simulink model "ElevatorPlant_Storage_A"  (R2015b)
(part 8 of 8)

            state First_but_3
              en:
              BUT_1=BUT_TEMP;
              FIRST_BUT=false;
            (default) -> (junction 79574)
            (junction 79574) -> Emergency.Doors.Closing2.Button_detection.BUTTON_DOWN.Button_DOWN_1 [order 1] : [PD1]
            Emergency.Doors.Closing2.Button_detection.BUTTON_DOWN.Button_DOWN_1 -> (junction 79575)
            (junction 79575) -> Emergency.Doors.Closing2.Button_detection.BUTTON_DOWN.First_but_1 [order 1] : [FIRST_BUT && not(RPC1)]
            Emergency.Doors.Closing2.Button_detection.BUTTON_DOWN.First_but_1 -> (junction 79576)
            (junction 79574) -> (junction 79577) [order 2]
            (junction 79575) -> (junction 79578) [order 2]
            (junction 79576) -> (junction 79579)
            (junction 79578) -> (junction 79577)
            (junction 79579) -> (junction 79578)
            (junction 79577) -> (junction 79580)
            (junction 79580) -> Emergency.Doors.Closing2.Button_detection.BUTTON_DOWN.Button_DOWN_2 [order 1] : [PD2]
            Emergency.Doors.Closing2.Button_detection.BUTTON_DOWN.Button_DOWN_2 -> (junction 79581)
            (junction 79581) -> Emergency.Doors.Closing2.Button_detection.BUTTON_DOWN.First_but_2 [order 1] : [FIRST_BUT && not(RPC2)]
            Emergency.Doors.Closing2.Button_detection.BUTTON_DOWN.First_but_2 -> (junction 79582)
            (junction 79580) -> (junction 79583) [order 2]
            (junction 79581) -> (junction 79584) [order 2]
            (junction 79582) -> (junction 79585)
            (junction 79584) -> (junction 79583)
            (junction 79585) -> (junction 79584)
            (junction 79583) -> (junction 79586)
            (junction 79586) -> Emergency.Doors.Closing2.Button_detection.BUTTON_DOWN.Button_DOWN_3 [order 1] : [PD3]
            Emergency.Doors.Closing2.Button_detection.BUTTON_DOWN.Button_DOWN_3 -> (junction 79587)
            (junction 79587) -> Emergency.Doors.Closing2.Button_detection.BUTTON_DOWN.First_but_3 [order 1] : [FIRST_BUT && not(RPC3)]
            Emergency.Doors.Closing2.Button_detection.BUTTON_DOWN.First_but_3 -> (junction 79588)
            (junction 79586) -> (junction 79589) [order 2]
            (junction 79587) -> (junction 79590) [order 2]
            (junction 79588) -> (junction 79591)
            (junction 79590) -> (junction 79589)
            (junction 79591) -> (junction 79590)
          state BUTTON_CAR
            state Button_CAR_0
              en:
              BUTTON_CAR(1)=true;
              BUT_TEMP=0;
              LPC0=true;
              PUSHED=true;
              UPDATE=false;
              IN_LL=false; ET_LL=0;
            state First_but_0
              en:
              BUT_1=BUT_TEMP;
              FIRST_BUT=false;
            state Button_CAR_1
              en:
              BUTTON_CAR(2)=true;
              BUT_TEMP=1;
              LPC1=true;
              PUSHED=true;
              UPDATE=false;
              IN_LL=false; ET_LL=0;
            state First_but_1
              en:
              BUT_1=BUT_TEMP;
              FIRST_BUT=false;
            state Button_CAR_2
              en:
              BUTTON_CAR(3)=true;
              BUT_TEMP=2;
              LPC2=true;
              PUSHED=true;
              UPDATE=false;
              IN_LL=false; ET_LL=0;
            state First_but_2
              en:
              BUT_1=BUT_TEMP;
              FIRST_BUT=false;
            state Button_CAR_3
              en:
              BUTTON_CAR(4)=true;
              BUT_TEMP=3;
              LPC3=true;
              PUSHED=true;
              UPDATE=false;
              IN_LL=false; ET_LL=0;
            state First_but_3
              en:
              BUT_1=BUT_TEMP;
              FIRST_BUT=false;
            (default) -> (junction 79629)
            (junction 79629) -> Emergency.Doors.Closing2.Button_detection.BUTTON_CAR.Button_CAR_0 [order 1] : [P0]
            Emergency.Doors.Closing2.Button_detection.BUTTON_CAR.Button_CAR_0 -> (junction 79630)
            (junction 79630) -> Emergency.Doors.Closing2.Button_detection.BUTTON_CAR.First_but_0 [order 1] : [FIRST_BUT && not(RPC0)]
            Emergency.Doors.Closing2.Button_detection.BUTTON_CAR.First_but_0 -> (junction 79631)
            (junction 79629) -> (junction 79632) [order 2]
            (junction 79630) -> (junction 79633) [order 2]
            (junction 79631) -> (junction 79634)
            (junction 79633) -> (junction 79632)
            (junction 79634) -> (junction 79633)
            (junction 79632) -> (junction 79637)
            Emergency.Doors.Closing2.Button_detection.BUTTON_CAR.Button_CAR_1 -> (junction 79635)
            (junction 79635) -> Emergency.Doors.Closing2.Button_detection.BUTTON_CAR.First_but_1 [order 1] : [FIRST_BUT && not(RPC1)]
            Emergency.Doors.Closing2.Button_detection.BUTTON_CAR.First_but_1 -> (junction 79636)
            (junction 79635) -> (junction 79639) [order 2]
            (junction 79636) -> (junction 79640)
            (junction 79637) -> Emergency.Doors.Closing2.Button_detection.BUTTON_CAR.Button_CAR_1 [order 1] : [P1]
            (junction 79637) -> (junction 79638) [order 2]
            (junction 79639) -> (junction 79638)
            (junction 79640) -> (junction 79639)
            (junction 79638) -> (junction 79641)
            (junction 79641) -> Emergency.Doors.Closing2.Button_detection.BUTTON_CAR.Button_CAR_2 [order 1] : [P2]
            Emergency.Doors.Closing2.Button_detection.BUTTON_CAR.Button_CAR_2 -> (junction 79642)
            (junction 79642) -> Emergency.Doors.Closing2.Button_detection.BUTTON_CAR.First_but_2 [order 1] : [FIRST_BUT && not(RPC2)]
            Emergency.Doors.Closing2.Button_detection.BUTTON_CAR.First_but_2 -> (junction 79643)
            (junction 79641) -> (junction 79644) [order 2]
            (junction 79642) -> (junction 79645) [order 2]
            (junction 79643) -> (junction 79646)
            (junction 79645) -> (junction 79644)
            (junction 79646) -> (junction 79645)
            (junction 79644) -> (junction 79647)
            (junction 79647) -> Emergency.Doors.Closing2.Button_detection.BUTTON_CAR.Button_CAR_3 [order 1] : [P3]
            Emergency.Doors.Closing2.Button_detection.BUTTON_CAR.Button_CAR_3 -> (junction 79648)
            (junction 79648) -> Emergency.Doors.Closing2.Button_detection.BUTTON_CAR.First_but_3 [order 1] : [FIRST_BUT && not(RPC3)]
            Emergency.Doors.Closing2.Button_detection.BUTTON_CAR.First_but_3 -> (junction 79649)
            (junction 79647) -> (junction 79650) [order 2]
            (junction 79648) -> (junction 79651) [order 2]
            (junction 79649) -> (junction 79652)
            (junction 79651) -> (junction 79650)
            (junction 79652) -> (junction 79651)
          state BUTTON_UP
            state Button_UP_0
              en:
              BUTTON_UP(1)=true;
              BUT_TEMP=0;
              LPS0=true;
              PUSHED=true;
              UPDATE=false;
              IN_LL=false; ET_LL=0;
            state First_but_0
              en:
              BUT_1=BUT_TEMP;
              FIRST_BUT=false;
            state Button_UP_1
              en:
              BUTTON_UP(2)=true;
              BUT_TEMP=1;
              LPS1=true;
              PUSHED=true;
              UPDATE=false;
              IN_LL=false; ET_LL=0;
            state First_but_1
              en:
              BUT_1=BUT_TEMP;
              FIRST_BUT=false;
            state Button_UP_2
              en:
              BUTTON_UP(3)=true;
              BUT_TEMP=2;
              LPS2=true;
              PUSHED=true;
              UPDATE=false;
              IN_LL=false; ET_LL=0;
            state First_but_2
              en:
              BUT_1=BUT_TEMP;
              FIRST_BUT=false;
            (junction 79702) -> Emergency.Doors.Closing2.Button_detection.BUTTON_UP.Button_UP_0 [order 1] : [PS0]
            Emergency.Doors.Closing2.Button_detection.BUTTON_UP.Button_UP_0 -> (junction 79703)
            (junction 79703) -> Emergency.Doors.Closing2.Button_detection.BUTTON_UP.First_but_0 [order 1] : [FIRST_BUT && not(RPC0)]
            Emergency.Doors.Closing2.Button_detection.BUTTON_UP.First_but_0 -> (junction 79704)
            (default) -> (junction 79702)
            (junction 79702) -> (junction 79707) [order 2]
            (junction 79703) -> (junction 79705) [order 2]
            (junction 79704) -> (junction 79706)
            (junction 79706) -> (junction 79705)
            (junction 79705) -> (junction 79707)
            (junction 79707) -> (junction 79708)
            (junction 79708) -> Emergency.Doors.Closing2.Button_detection.BUTTON_UP.Button_UP_1 [order 1] : [PS1]
            Emergency.Doors.Closing2.Button_detection.BUTTON_UP.Button_UP_1 -> (junction 79709)
            (junction 79709) -> Emergency.Doors.Closing2.Button_detection.BUTTON_UP.First_but_1 [order 1] : [FIRST_BUT && not(RPC1)]
            Emergency.Doors.Closing2.Button_detection.BUTTON_UP.First_but_1 -> (junction 79710)
            (junction 79708) -> (junction 79711) [order 2]
            (junction 79709) -> (junction 79712) [order 2]
            (junction 79710) -> (junction 79713)
            (junction 79712) -> (junction 79711)
            (junction 79713) -> (junction 79712)
            (junction 79711) -> (junction 79715)
            Emergency.Doors.Closing2.Button_detection.BUTTON_UP.First_but_2 -> (junction 79714)
            (junction 79714) -> (junction 79719)
            (junction 79715) -> Emergency.Doors.Closing2.Button_detection.BUTTON_UP.Button_UP_2 [order 1] : [PS2]
            Emergency.Doors.Closing2.Button_detection.BUTTON_UP.Button_UP_2 -> (junction 79716)
            (junction 79716) -> Emergency.Doors.Closing2.Button_detection.BUTTON_UP.First_but_2 [order 1] : [FIRST_BUT && not(RPC2)]
            (junction 79715) -> (junction 79717) [order 2]
            (junction 79716) -> (junction 79718) [order 2]
            (junction 79718) -> (junction 79717)
            (junction 79719) -> (junction 79718)
          state Max_Min_assignment
            state Min_but
              en:
              BUTTON=MIN_BUT;
            state Max_but
              en:
              BUTTON=MAX_BUT;
            state First_but
              en:
              BUTTON=BUT_1;
            state Max_but1
              en:
              MAX_BUT=2;
            state Max_but2
              en:
              MAX_BUT=1;
            state Max_but3
              en:
              MAX_BUT=0;
            state Min_but1
              en:
              MIN_BUT=1;
            state Min_but2
              en:
              MIN_BUT=2;
            state Min_but3
              en:
              MIN_BUT=3;
            state MAX
              en:
              MAX_BUT=BUT_TEMP;
            state MIN
              en:
              MIN_BUT=BUT_TEMP;
            state Updating_button_0
              en:
              BUTTON=MAX_BUT;
            state Updating_button_1
              en:
              BUTTON=MIN_BUT;
            (junction 79757) -> Emergency.Doors.Closing2.Button_detection.Max_Min_assignment.Min_but [order 1] : [(MAX_BUT-FLOOR)>(FLOOR-MIN_BUT)]
            Emergency.Doors.Closing2.Button_detection.Max_Min_assignment.Min_but -> (junction 79758)
            (junction 79759) -> (junction 79757) [order 1] : [not(FLAG_STOP) && MOTION==2 && FLAG==3]
            (default) -> (junction 79759)
            (junction 79757) -> (junction 79760) [order 2]
            (junction 79758) -> (junction 79761)
            (junction 79759) -> (junction 79762) [order 2]
            (junction 79760) -> Emergency.Doors.Closing2.Button_detection.Max_Min_assignment.Max_but [order 1] : [(MAX_BUT-FLOOR)<(FLOOR-MIN_BUT)]
            Emergency.Doors.Closing2.Button_detection.Max_Min_assignment.Max_but -> (junction 79761)
            (junction 79760) -> Emergency.Doors.Closing2.Button_detection.Max_Min_assignment.First_but [order 2]
            (junction 79761) -> (junction 79764)
            Emergency.Doors.Closing2.Button_detection.Max_Min_assignment.First_but -> (junction 79763)
            (junction 79763) -> (junction 79762)
            (junction 79764) -> (junction 79763)
            (junction 79762) -> (junction 79765)
            (junction 79766) -> (junction 79767) [order 1] : [MOTION==0]
                | {MOTION=1;
                | UPDATE=true;}
            (junction 79767) -> Emergency.Doors.Closing2.Button_detection.Max_Min_assignment.Max_but1 [order 1] : [BUTTON_UP(2)]
            Emergency.Doors.Closing2.Button_detection.Max_Min_assignment.Max_but1 -> (junction 79768)
            (junction 79765) -> (junction 79766) [order 1] : [BUTTON==FLOOR && EXTEND]
                | {EXTEND=false;}
            (junction 79765) -> (junction 79779) [order 2]
            (junction 79766) -> (junction 79771) [order 2]
            (junction 79767) -> (junction 79769) [order 2]
            (junction 79768) -> (junction 79770)
            (junction 79769) -> Emergency.Doors.Closing2.Button_detection.Max_Min_assignment.Max_but2 [order 1] : [BUTTON_UP(1)]
            Emergency.Doors.Closing2.Button_detection.Max_Min_assignment.Max_but2 -> (junction 79770)
            (junction 79769) -> Emergency.Doors.Closing2.Button_detection.Max_Min_assignment.Max_but3 [order 2]
            (junction 79770) -> (junction 79773)
            Emergency.Doors.Closing2.Button_detection.Max_Min_assignment.Max_but3 -> (junction 79772)
            (junction 79772) -> (junction 79771)
            (junction 79773) -> (junction 79772)
            (junction 79771) -> (junction 79774)
            (junction 79774) -> (junction 79775) [order 1] : [MOTION==1]
                | {MOTION=0;
                | UPDATE=true;}
            (junction 79775) -> Emergency.Doors.Closing2.Button_detection.Max_Min_assignment.Min_but1 [order 1] : [BUTTON_DOWN(1)]
            Emergency.Doors.Closing2.Button_detection.Max_Min_assignment.Min_but1 -> (junction 79776)
            (junction 79774) -> (junction 79780) [order 2]
            (junction 79775) -> (junction 79777) [order 2]
            (junction 79776) -> (junction 79778)
            (junction 79777) -> Emergency.Doors.Closing2.Button_detection.Max_Min_assignment.Min_but2 [order 1] : [BUTTON_DOWN(2)]
            Emergency.Doors.Closing2.Button_detection.Max_Min_assignment.Min_but2 -> (junction 79778)
            (junction 79777) -> Emergency.Doors.Closing2.Button_detection.Max_Min_assignment.Min_but3 [order 2]
            (junction 79778) -> (junction 79782)
            Emergency.Doors.Closing2.Button_detection.Max_Min_assignment.Min_but3 -> (junction 79781)
            (junction 79780) -> (junction 79779)
            (junction 79781) -> (junction 79780)
            (junction 79782) -> (junction 79781)
            (junction 79779) -> (junction 79784)
            Emergency.Doors.Closing2.Button_detection.Max_Min_assignment.MAX -> (junction 79783)
            (junction 79784) -> (junction 79785) [order 1] : [PUSHED]
            (junction 79785) -> (junction 79786) [order 1] : [not(BUT_TEMP==FLOOR) || not(MOTION==2)]
            (junction 79786) -> Emergency.Doors.Closing2.Button_detection.Max_Min_assignment.MAX [order 1] : [MAX_BUT<BUT_TEMP && not(UPDATE)]
            (junction 79783) -> (junction 79788)
            (junction 79784) -> (junction 79798) [order 2]
            (junction 79785) -> (junction 79791) [order 2]
            (junction 79786) -> (junction 79787) [order 2]
            (junction 79788) -> (junction 79787)
            (junction 79787) -> (junction 79789)
            (junction 79789) -> Emergency.Doors.Closing2.Button_detection.Max_Min_assignment.MIN [order 1] : [MIN_BUT>BUT_TEMP && not(UPDATE)]
            Emergency.Doors.Closing2.Button_detection.Max_Min_assignment.MIN -> (junction 79790)
            (junction 79789) -> (junction 79792) [order 2]
            (junction 79790) -> (junction 79793)
            (junction 79792) -> (junction 79791)
            (junction 79793) -> (junction 79792)
            (junction 79791) -> (junction 79794)
            (junction 79794) -> Emergency.Doors.Closing2.Button_detection.Max_Min_assignment.Updating_button_0 [order 1] : [MOTION==0]
            Emergency.Doors.Closing2.Button_detection.Max_Min_assignment.Updating_button_0 -> (junction 79795)
            (junction 79794) -> (junction 79796) [order 2]
            (junction 79795) -> (junction 79797)
            (junction 79796) -> Emergency.Doors.Closing2.Button_detection.Max_Min_assignment.Updating_button_1 [order 1] : [MOTION==1]
            Emergency.Doors.Closing2.Button_detection.Max_Min_assignment.Updating_button_1 -> (junction 79797)
            (junction 79796) -> (junction 79799) [order 2]
            (junction 79797) -> (junction 79800)
            (junction 79799) -> (junction 79798)
            (junction 79800) -> (junction 79799)
          state GoTo_PositionControl
            en:
            BUTTON=BUT_TEMP;
            FLAG=2;
          state Emergency
            en:
            FLAG_EMG=true;
            FLAG=4;
          state Timer_EME
            state Set_tmr
              en:
              Q_EME=true;
            state Counting
              en:
              ET_EME= ET_EME + 1;
              Q_EME=false;
            state Set
              en:
              IN_EME=true;
              PT_EME=3;
            (junction 79890) -> Emergency.Doors.Closing2.Button_detection.Timer_EME.Set_tmr [order 1] : [ET_EME==PT_EME]
            Emergency.Doors.Closing2.Button_detection.Timer_EME.Set_tmr -> (junction 79891)
            Emergency.Doors.Closing2.Button_detection.Timer_EME.Counting -> (junction 79890)
            (junction 79890) -> (junction 79891) [order 2]
            (default) -> Emergency.Doors.Closing2.Button_detection.Timer_EME.Set
            Emergency.Doors.Closing2.Button_detection.Timer_EME.Set -> (junction 79892)
            (junction 79892) -> Emergency.Doors.Closing2.Button_detection.Timer_EME.Counting [order 1] : [ET_EME<PT_EME]
            (junction 79892) -> (junction 79891) [order 2]
          state Not_Emergency
            en:
            IN_EME=false;
            ET_EME=0;
          state SwitchingOFF_LEDs
            en:
            LPD3=false;
            LPD2=false;
            LPS2=false;
            LPD1=false;
            LPS1=false;
            LPS0=false;
          (default) -> (junction 79491)
          (junction 79491) -> (junction 79492) [order 1] : [FLAG==1 && not(PUSHED)]
              | {BUTTON=FLOOR;
              | BUT_TEMP=BUTTON;
              | BUT_1=FLOOR;}
          (junction 79492) -> Emergency.Doors.Closing2.Button_detection.Timer_LL [order 1] : [not(FLAG_STOP)]
          Emergency.Doors.Closing2.Button_detection.Save_energy -> (junction 79493)
          Emergency.Doors.Closing2.Button_detection.Timer_LL -> Emergency.Doors.Closing2.Button_detection.Save_energy
          (junction 79492) -> (junction 79495) [order 2]
          (junction 79491) -> (junction 79494) [order 2]
          (junction 79493) -> (junction 79496)
          (junction 79495) -> (junction 79494)
          (junction 79496) -> (junction 79495)
          (junction 79494) -> Emergency.Doors.Closing2.Button_detection.BUTTON_CAR
          Emergency.Doors.Closing2.Button_detection.BUTTON_UP -> Emergency.Doors.Closing2.Button_detection.BUTTON_DOWN
          Emergency.Doors.Closing2.Button_detection.BUTTON_DOWN -> Emergency.Doors.Closing2.Button_detection.Max_Min_assignment
          Emergency.Doors.Closing2.Button_detection.Max_Min_assignment -> (junction 79497)
          Emergency.Doors.Closing2.Button_detection.BUTTON_CAR -> Emergency.Doors.Closing2.Button_detection.BUTTON_UP
          (junction 79497) -> (junction 79499)
          (junction 79499) -> (junction 79498)
          (junction 79498) -> (junction 79501)
          Emergency.Doors.Closing2.Button_detection.GoTo_PositionControl -> (junction 79500)
          (junction 79501) -> (junction 79502) [order 1] : [FLAG==1]
          (junction 79502) -> Emergency.Doors.Closing2.Button_detection.GoTo_PositionControl [order 1] : [PUSHED]
          (junction 79500) -> (junction 79504)
          (junction 79501) -> (junction 79512) [order 2]
          (junction 79502) -> (junction 79503) [order 2]
          (junction 79504) -> (junction 79503)
          (junction 79503) -> (junction 79506)
          Emergency.Doors.Closing2.Button_detection.Emergency -> (junction 79505)
          (junction 79506) -> Emergency.Doors.Closing2.Button_detection.Timer_EME [order 1] : [STOP]
              | {IN_LL=false; ET_LL=0;FLAG=1;}
          Emergency.Doors.Closing2.Button_detection.Timer_EME -> (junction 79507)
          (junction 79507) -> Emergency.Doors.Closing2.Button_detection.Emergency [order 1] : [Q_EME]
          (junction 79505) -> (junction 79509)
          (junction 79506) -> Emergency.Doors.Closing2.Button_detection.Not_Emergency [order 2]
          (junction 79507) -> (junction 79508) [order 2]
          (junction 79509) -> (junction 79508)
          (junction 79508) -> (junction 79511)
          Emergency.Doors.Closing2.Button_detection.Not_Emergency -> (junction 79511)
          Emergency.Doors.Closing2.Button_detection.SwitchingOFF_LEDs -> (junction 79510)
          (junction 79511) -> Emergency.Doors.Closing2.Button_detection.SwitchingOFF_LEDs [order 1] : [FLAG_STOP && FLAG==2]
          (junction 79510) -> (junction 79514)
          (junction 79511) -> (junction 79513) [order 2]
          (junction 79513) -> (junction 79512)
          (junction 79514) -> (junction 79513)
        state Extending
          en:
          EXTEND=true;
        state Stop_Closing
          en:
          CP2=false;
          FLAG_OD=false;
          OBS=false;
          ET_cl=0;
          IN_cl=false;
        state GoTo_PositionControl
          en: FLAG=2;
        state GoTo_BUttonDetection
          en:
          MOTION=2;
          MAX_BUT=0;
          MIN_BUT=3;
          PUSHED=false;
          FIRST_BUT=true;
          FLAG=1;
          UPDATE=false;
        state Closing1
          en:CP2=true;
        state Stop_Closing1
          en:CP2=false;
        Emergency.Doors.Closing2.Reset -> Emergency.Doors.Closing2.Timer_close
        (default) -> (junction 79402)
        (junction 79402) -> Emergency.Doors.Closing2.Reset [order 1] : [not(FLAG==0) && not(FLAG==4)]
        Emergency.Doors.Closing2.Timer_close -> (junction 79403)
        (junction 79403) -> Emergency.Doors.Closing2.Closing [order 1] : [not(PC2)]
        Emergency.Doors.Closing2.Button_detection -> (junction 79404)
        Emergency.Doors.Closing2.Closing -> Emergency.Doors.Closing2.Button_detection
        (junction 79402) -> (junction 79412) [order 2]
        (junction 79403) -> (junction 79405) [order 2]
        (junction 79404) -> (junction 79410)
        (junction 79405) -> Emergency.Doors.Closing2.Extending [order 1] : [BUTTON==FLOOR]
        (junction 79405) -> (junction 79407) [order 2]
        Emergency.Doors.Closing2.Extending -> (junction 79406)
        (junction 79406) -> (junction 79407)
        (junction 79407) -> Emergency.Doors.Closing2.Stop_Closing
        Emergency.Doors.Closing2.Stop_Closing -> (junction 79408)
        (junction 79408) -> Emergency.Doors.Closing2.GoTo_PositionControl [order 2]
        (junction 79408) -> Emergency.Doors.Closing2.GoTo_BUttonDetection [order 1] : [not(BUTTON_CAR(1) || BUTTON_CAR(2) || BUTTON_CAR(3) || BUTTON_CAR(4) || BUTTON_UP(1) || BUTTON_UP(2) || BUTTON_UP(3) || BUTTON_DOWN(2) || BUTTON_DOWN(3) || BUTTON_DOWN(4))]
        Emergency.Doors.Closing2.GoTo_PositionControl -> (junction 79409)
        Emergency.Doors.Closing2.GoTo_BUttonDetection -> (junction 79409)
        (junction 79409) -> (junction 79410)
        (junction 79410) -> (junction 79411)
        (junction 79411) -> (junction 79413)
        (junction 79412) -> Emergency.Doors.Closing2.Closing1 [order 1] : [not(PC2)]
        Emergency.Doors.Closing2.Closing1 -> (junction 79413)
        (junction 79412) -> Emergency.Doors.Closing2.Stop_Closing1 [order 2]
        Emergency.Doors.Closing2.Stop_Closing1 -> (junction 79413)
      state Closing3
        state Reset
          state Reset_0
            en:
            LPS0=false;
            BUTTON_CAR(1)=false;
            BUTTON_UP(1)=false;
          state Reset_1
            en:
            LPS1=false;
            LPD1=false;
            BUTTON_CAR(2)=false;
            BUTTON_UP(2)=false;
            BUTTON_DOWN(2)=false;
          state Reset_2
            en:
            LPS2=false;
            LPD2=false;
            BUTTON_CAR(3)=false;
            BUTTON_UP(3)=false;
            BUTTON_DOWN(3)=false;
          state Reset_3
            en:
            LPD3=false;
            BUTTON_CAR(4)=false;
            BUTTON_DOWN(4)=false;
          (default) -> (junction 79953)
          (junction 79953) -> Emergency.Doors.Closing3.Reset.Reset_0 [order 1] : [FLOOR==0]
          Emergency.Doors.Closing3.Reset.Reset_0 -> (junction 79954)
          (junction 79953) -> (junction 79955) [order 2]
          (junction 79954) -> (junction 79956)
          (junction 79955) -> Emergency.Doors.Closing3.Reset.Reset_1 [order 1] : [FLOOR==1]
          Emergency.Doors.Closing3.Reset.Reset_1 -> (junction 79956)
          (junction 79955) -> (junction 79957) [order 2]
          (junction 79956) -> (junction 79958)
          (junction 79957) -> Emergency.Doors.Closing3.Reset.Reset_2 [order 1] : [FLOOR==2]
          Emergency.Doors.Closing3.Reset.Reset_2 -> (junction 79958)
          (junction 79957) -> (junction 79959) [order 2]
          (junction 79958) -> (junction 79960)
          (junction 79959) -> Emergency.Doors.Closing3.Reset.Reset_3 [order 1] : [FLOOR==3]
          Emergency.Doors.Closing3.Reset.Reset_3 -> (junction 79960)
          (junction 79959) -> (junction 79961) [order 2]
          (junction 79960) -> (junction 79962)
          (junction 79962) -> (junction 79961)
        state Timer_close
          state Set_tmr
            en: Q_cl=true;
          state Set
            en:PT_cl=5;
            IN_cl=true;
          state Counting
            en:ET_cl = ET_cl + 1;
            Q_cl=false;
          (junction 79986) -> Emergency.Doors.Closing3.Timer_close.Set_tmr [order 1] : [ET_cl==PT_cl]
          Emergency.Doors.Closing3.Timer_close.Set_tmr -> (junction 79987)
          (default) -> Emergency.Doors.Closing3.Timer_close.Set
          Emergency.Doors.Closing3.Timer_close.Counting -> (junction 79986)
          (junction 79986) -> (junction 79987) [order 2]
          Emergency.Doors.Closing3.Timer_close.Set -> (junction 79988)
          (junction 79988) -> Emergency.Doors.Closing3.Timer_close.Counting [order 1] : [ET_cl<PT_cl]
          (junction 79988) -> (junction 79987) [order 2]
        state Closing
          en: CP2=Q_cl;
        state Button_detection
          state Save_energy
            en:
            LL=not(Q_LL);
          state Timer_LL
            state Set_tmr
              en:
              Q_LL=true;
            state Counting
              en:
              ET_LL= ET_LL + 1;
              Q_LL=false;
            state Set
              en:
              IN_LL=true;
              PT_LL=10;
            (junction 80070) -> Emergency.Doors.Closing3.Button_detection.Timer_LL.Set_tmr [order 1] : [ET_LL==PT_LL]
            Emergency.Doors.Closing3.Button_detection.Timer_LL.Set_tmr -> (junction 80071)
            Emergency.Doors.Closing3.Button_detection.Timer_LL.Counting -> (junction 80070)
            (junction 80070) -> (junction 80071) [order 2]
            (default) -> Emergency.Doors.Closing3.Button_detection.Timer_LL.Set
            Emergency.Doors.Closing3.Button_detection.Timer_LL.Set -> (junction 80072)
            (junction 80072) -> Emergency.Doors.Closing3.Button_detection.Timer_LL.Counting [order 1] : [ET_LL<PT_LL]
            (junction 80072) -> (junction 80071) [order 2]
          state BUTTON_DOWN
            state Button_DOWN_1
              en:
              BUTTON_DOWN(2)=true;
              BUT_TEMP=1;
              LPD1=true;
              PUSHED=true;
              UPDATE=false;
              IN_LL=false; ET_LL=0;
            state First_but_1
              en:
              BUT_1=BUT_TEMP;
              FIRST_BUT=false;
            state Button_DOWN_2
              en:
              BUTTON_DOWN(3)=true;
              BUT_TEMP=2;
              LPD2=true;
              PUSHED=true;
              UPDATE=false;
              IN_LL=false; ET_LL=0;
            state First_but_2
              en:
              BUT_1=BUT_TEMP;
              FIRST_BUT=false;
            state Button_DOWN_3
              en:
              BUTTON_DOWN(4)=true;
              BUT_TEMP=3;
              LPD3=true;
              PUSHED=true;
              UPDATE=false;
              IN_LL=false; ET_LL=0;
            state First_but_3
              en:
              BUT_1=BUT_TEMP;
              FIRST_BUT=false;
            (default) -> (junction 80085)
            (junction 80085) -> Emergency.Doors.Closing3.Button_detection.BUTTON_DOWN.Button_DOWN_1 [order 1] : [PD1]
            Emergency.Doors.Closing3.Button_detection.BUTTON_DOWN.Button_DOWN_1 -> (junction 80086)
            (junction 80086) -> Emergency.Doors.Closing3.Button_detection.BUTTON_DOWN.First_but_1 [order 1] : [FIRST_BUT && not(RPC1)]
            Emergency.Doors.Closing3.Button_detection.BUTTON_DOWN.First_but_1 -> (junction 80087)
            (junction 80085) -> (junction 80088) [order 2]
            (junction 80086) -> (junction 80089) [order 2]
            (junction 80087) -> (junction 80090)
            (junction 80089) -> (junction 80088)
            (junction 80090) -> (junction 80089)
            (junction 80088) -> (junction 80091)
            (junction 80091) -> Emergency.Doors.Closing3.Button_detection.BUTTON_DOWN.Button_DOWN_2 [order 1] : [PD2]
            Emergency.Doors.Closing3.Button_detection.BUTTON_DOWN.Button_DOWN_2 -> (junction 80092)
            (junction 80092) -> Emergency.Doors.Closing3.Button_detection.BUTTON_DOWN.First_but_2 [order 1] : [FIRST_BUT && not(RPC2)]
            Emergency.Doors.Closing3.Button_detection.BUTTON_DOWN.First_but_2 -> (junction 80093)
            (junction 80091) -> (junction 80094) [order 2]
            (junction 80092) -> (junction 80095) [order 2]
            (junction 80093) -> (junction 80096)
            (junction 80095) -> (junction 80094)
            (junction 80096) -> (junction 80095)
            (junction 80094) -> (junction 80097)
            (junction 80097) -> Emergency.Doors.Closing3.Button_detection.BUTTON_DOWN.Button_DOWN_3 [order 1] : [PD3]
            Emergency.Doors.Closing3.Button_detection.BUTTON_DOWN.Button_DOWN_3 -> (junction 80098)
            (junction 80098) -> Emergency.Doors.Closing3.Button_detection.BUTTON_DOWN.First_but_3 [order 1] : [FIRST_BUT && not(RPC3)]
            Emergency.Doors.Closing3.Button_detection.BUTTON_DOWN.First_but_3 -> (junction 80099)
            (junction 80097) -> (junction 80100) [order 2]
            (junction 80098) -> (junction 80101) [order 2]
            (junction 80099) -> (junction 80102)
            (junction 80101) -> (junction 80100)
            (junction 80102) -> (junction 80101)
          state BUTTON_CAR
            state Button_CAR_0
              en:
              BUTTON_CAR(1)=true;
              BUT_TEMP=0;
              LPC0=true;
              PUSHED=true;
              UPDATE=false;
              IN_LL=false; ET_LL=0;
            state First_but_0
              en:
              BUT_1=BUT_TEMP;
              FIRST_BUT=false;
            state Button_CAR_1
              en:
              BUTTON_CAR(2)=true;
              BUT_TEMP=1;
              LPC1=true;
              PUSHED=true;
              UPDATE=false;
              IN_LL=false; ET_LL=0;
            state First_but_1
              en:
              BUT_1=BUT_TEMP;
              FIRST_BUT=false;
            state Button_CAR_2
              en:
              BUTTON_CAR(3)=true;
              BUT_TEMP=2;
              LPC2=true;
              PUSHED=true;
              UPDATE=false;
              IN_LL=false; ET_LL=0;
            state First_but_2
              en:
              BUT_1=BUT_TEMP;
              FIRST_BUT=false;
            state Button_CAR_3
              en:
              BUTTON_CAR(4)=true;
              BUT_TEMP=3;
              LPC3=true;
              PUSHED=true;
              UPDATE=false;
              IN_LL=false; ET_LL=0;
            state First_but_3
              en:
              BUT_1=BUT_TEMP;
              FIRST_BUT=false;
            (default) -> (junction 80140)
            (junction 80140) -> Emergency.Doors.Closing3.Button_detection.BUTTON_CAR.Button_CAR_0 [order 1] : [P0]
            Emergency.Doors.Closing3.Button_detection.BUTTON_CAR.Button_CAR_0 -> (junction 80141)
            (junction 80141) -> Emergency.Doors.Closing3.Button_detection.BUTTON_CAR.First_but_0 [order 1] : [FIRST_BUT && not(RPC0)]
            Emergency.Doors.Closing3.Button_detection.BUTTON_CAR.First_but_0 -> (junction 80142)
            (junction 80140) -> (junction 80143) [order 2]
            (junction 80141) -> (junction 80144) [order 2]
            (junction 80142) -> (junction 80145)
            (junction 80144) -> (junction 80143)
            (junction 80145) -> (junction 80144)
            (junction 80143) -> (junction 80148)
            Emergency.Doors.Closing3.Button_detection.BUTTON_CAR.Button_CAR_1 -> (junction 80146)
            (junction 80146) -> Emergency.Doors.Closing3.Button_detection.BUTTON_CAR.First_but_1 [order 1] : [FIRST_BUT && not(RPC1)]
            Emergency.Doors.Closing3.Button_detection.BUTTON_CAR.First_but_1 -> (junction 80147)
            (junction 80146) -> (junction 80150) [order 2]
            (junction 80147) -> (junction 80151)
            (junction 80148) -> Emergency.Doors.Closing3.Button_detection.BUTTON_CAR.Button_CAR_1 [order 1] : [P1]
            (junction 80148) -> (junction 80149) [order 2]
            (junction 80150) -> (junction 80149)
            (junction 80151) -> (junction 80150)
            (junction 80149) -> (junction 80152)
            (junction 80152) -> Emergency.Doors.Closing3.Button_detection.BUTTON_CAR.Button_CAR_2 [order 1] : [P2]
            Emergency.Doors.Closing3.Button_detection.BUTTON_CAR.Button_CAR_2 -> (junction 80153)
            (junction 80153) -> Emergency.Doors.Closing3.Button_detection.BUTTON_CAR.First_but_2 [order 1] : [FIRST_BUT && not(RPC2)]
            Emergency.Doors.Closing3.Button_detection.BUTTON_CAR.First_but_2 -> (junction 80154)
            (junction 80152) -> (junction 80155) [order 2]
            (junction 80153) -> (junction 80156) [order 2]
            (junction 80154) -> (junction 80157)
            (junction 80156) -> (junction 80155)
            (junction 80157) -> (junction 80156)
            (junction 80155) -> (junction 80158)
            (junction 80158) -> Emergency.Doors.Closing3.Button_detection.BUTTON_CAR.Button_CAR_3 [order 1] : [P3]
            Emergency.Doors.Closing3.Button_detection.BUTTON_CAR.Button_CAR_3 -> (junction 80159)
            (junction 80159) -> Emergency.Doors.Closing3.Button_detection.BUTTON_CAR.First_but_3 [order 1] : [FIRST_BUT && not(RPC3)]
            Emergency.Doors.Closing3.Button_detection.BUTTON_CAR.First_but_3 -> (junction 80160)
            (junction 80158) -> (junction 80161) [order 2]
            (junction 80159) -> (junction 80162) [order 2]
            (junction 80160) -> (junction 80163)
            (junction 80162) -> (junction 80161)
            (junction 80163) -> (junction 80162)
          state BUTTON_UP
            state Button_UP_0
              en:
              BUTTON_UP(1)=true;
              BUT_TEMP=0;
              LPS0=true;
              PUSHED=true;
              UPDATE=false;
              IN_LL=false; ET_LL=0;
            state First_but_0
              en:
              BUT_1=BUT_TEMP;
              FIRST_BUT=false;
            state Button_UP_1
              en:
              BUTTON_UP(2)=true;
              BUT_TEMP=1;
              LPS1=true;
              PUSHED=true;
              UPDATE=false;
              IN_LL=false; ET_LL=0;
            state First_but_1
              en:
              BUT_1=BUT_TEMP;
              FIRST_BUT=false;
            state Button_UP_2
              en:
              BUTTON_UP(3)=true;
              BUT_TEMP=2;
              LPS2=true;
              PUSHED=true;
              UPDATE=false;
              IN_LL=false; ET_LL=0;
            state First_but_2
              en:
              BUT_1=BUT_TEMP;
              FIRST_BUT=false;
            (junction 80213) -> Emergency.Doors.Closing3.Button_detection.BUTTON_UP.Button_UP_0 [order 1] : [PS0]
            Emergency.Doors.Closing3.Button_detection.BUTTON_UP.Button_UP_0 -> (junction 80214)
            (junction 80214) -> Emergency.Doors.Closing3.Button_detection.BUTTON_UP.First_but_0 [order 1] : [FIRST_BUT && not(RPC0)]
            Emergency.Doors.Closing3.Button_detection.BUTTON_UP.First_but_0 -> (junction 80215)
            (default) -> (junction 80213)
            (junction 80213) -> (junction 80218) [order 2]
            (junction 80214) -> (junction 80216) [order 2]
            (junction 80215) -> (junction 80217)
            (junction 80217) -> (junction 80216)
            (junction 80216) -> (junction 80218)
            (junction 80218) -> (junction 80219)
            (junction 80219) -> Emergency.Doors.Closing3.Button_detection.BUTTON_UP.Button_UP_1 [order 1] : [PS1]
            Emergency.Doors.Closing3.Button_detection.BUTTON_UP.Button_UP_1 -> (junction 80220)
            (junction 80220) -> Emergency.Doors.Closing3.Button_detection.BUTTON_UP.First_but_1 [order 1] : [FIRST_BUT && not(RPC1)]
            Emergency.Doors.Closing3.Button_detection.BUTTON_UP.First_but_1 -> (junction 80221)
            (junction 80219) -> (junction 80222) [order 2]
            (junction 80220) -> (junction 80223) [order 2]
            (junction 80221) -> (junction 80224)
            (junction 80223) -> (junction 80222)
            (junction 80224) -> (junction 80223)
            (junction 80222) -> (junction 80226)
            Emergency.Doors.Closing3.Button_detection.BUTTON_UP.First_but_2 -> (junction 80225)
            (junction 80225) -> (junction 80230)
            (junction 80226) -> Emergency.Doors.Closing3.Button_detection.BUTTON_UP.Button_UP_2 [order 1] : [PS2]
            Emergency.Doors.Closing3.Button_detection.BUTTON_UP.Button_UP_2 -> (junction 80227)
            (junction 80227) -> Emergency.Doors.Closing3.Button_detection.BUTTON_UP.First_but_2 [order 1] : [FIRST_BUT && not(RPC2)]
            (junction 80226) -> (junction 80228) [order 2]
            (junction 80227) -> (junction 80229) [order 2]
            (junction 80229) -> (junction 80228)
            (junction 80230) -> (junction 80229)
          state Max_Min_assignment
            state Min_but
              en:
              BUTTON=MIN_BUT;
            state Max_but
              en:
              BUTTON=MAX_BUT;
            state First_but
              en:
              BUTTON=BUT_1;
            state Max_but1
              en:
              MAX_BUT=2;
            state Max_but2
              en:
              MAX_BUT=1;
            state Max_but3
              en:
              MAX_BUT=0;
            state Min_but1
              en:
              MIN_BUT=1;
            state Min_but2
              en:
              MIN_BUT=2;
            state Min_but3
              en:
              MIN_BUT=3;
            state MAX
              en:
              MAX_BUT=BUT_TEMP;
            state MIN
              en:
              MIN_BUT=BUT_TEMP;
            state Updating_button_0
              en:
              BUTTON=MAX_BUT;
            state Updating_button_1
              en:
              BUTTON=MIN_BUT;
            (junction 80268) -> Emergency.Doors.Closing3.Button_detection.Max_Min_assignment.Min_but [order 1] : [(MAX_BUT-FLOOR)>(FLOOR-MIN_BUT)]
            Emergency.Doors.Closing3.Button_detection.Max_Min_assignment.Min_but -> (junction 80269)
            (junction 80270) -> (junction 80268) [order 1] : [not(FLAG_STOP) && MOTION==2 && FLAG==3]
            (default) -> (junction 80270)
            (junction 80268) -> (junction 80271) [order 2]
            (junction 80269) -> (junction 80272)
            (junction 80270) -> (junction 80273) [order 2]
            (junction 80271) -> Emergency.Doors.Closing3.Button_detection.Max_Min_assignment.Max_but [order 1] : [(MAX_BUT-FLOOR)<(FLOOR-MIN_BUT)]
            Emergency.Doors.Closing3.Button_detection.Max_Min_assignment.Max_but -> (junction 80272)
            (junction 80271) -> Emergency.Doors.Closing3.Button_detection.Max_Min_assignment.First_but [order 2]
            (junction 80272) -> (junction 80275)
            Emergency.Doors.Closing3.Button_detection.Max_Min_assignment.First_but -> (junction 80274)
            (junction 80274) -> (junction 80273)
            (junction 80275) -> (junction 80274)
            (junction 80273) -> (junction 80276)
            (junction 80277) -> (junction 80278) [order 1] : [MOTION==0]
                | {MOTION=1;
                | UPDATE=true;}
            (junction 80278) -> Emergency.Doors.Closing3.Button_detection.Max_Min_assignment.Max_but1 [order 1] : [BUTTON_UP(2)]
            Emergency.Doors.Closing3.Button_detection.Max_Min_assignment.Max_but1 -> (junction 80279)
            (junction 80276) -> (junction 80277) [order 1] : [BUTTON==FLOOR && EXTEND]
                | {EXTEND=false;}
            (junction 80276) -> (junction 80290) [order 2]
            (junction 80277) -> (junction 80282) [order 2]
            (junction 80278) -> (junction 80280) [order 2]
            (junction 80279) -> (junction 80281)
            (junction 80280) -> Emergency.Doors.Closing3.Button_detection.Max_Min_assignment.Max_but2 [order 1] : [BUTTON_UP(1)]
            Emergency.Doors.Closing3.Button_detection.Max_Min_assignment.Max_but2 -> (junction 80281)
            (junction 80280) -> Emergency.Doors.Closing3.Button_detection.Max_Min_assignment.Max_but3 [order 2]
            (junction 80281) -> (junction 80284)
            Emergency.Doors.Closing3.Button_detection.Max_Min_assignment.Max_but3 -> (junction 80283)
            (junction 80283) -> (junction 80282)
            (junction 80284) -> (junction 80283)
            (junction 80282) -> (junction 80285)
            (junction 80285) -> (junction 80286) [order 1] : [MOTION==1]
                | {MOTION=0;
                | UPDATE=true;}
            (junction 80286) -> Emergency.Doors.Closing3.Button_detection.Max_Min_assignment.Min_but1 [order 1] : [BUTTON_DOWN(1)]
            Emergency.Doors.Closing3.Button_detection.Max_Min_assignment.Min_but1 -> (junction 80287)
            (junction 80285) -> (junction 80291) [order 2]
            (junction 80286) -> (junction 80288) [order 2]
            (junction 80287) -> (junction 80289)
            (junction 80288) -> Emergency.Doors.Closing3.Button_detection.Max_Min_assignment.Min_but2 [order 1] : [BUTTON_DOWN(2)]
            Emergency.Doors.Closing3.Button_detection.Max_Min_assignment.Min_but2 -> (junction 80289)
            (junction 80288) -> Emergency.Doors.Closing3.Button_detection.Max_Min_assignment.Min_but3 [order 2]
            (junction 80289) -> (junction 80293)
            Emergency.Doors.Closing3.Button_detection.Max_Min_assignment.Min_but3 -> (junction 80292)
            (junction 80291) -> (junction 80290)
            (junction 80292) -> (junction 80291)
            (junction 80293) -> (junction 80292)
            (junction 80290) -> (junction 80295)
            Emergency.Doors.Closing3.Button_detection.Max_Min_assignment.MAX -> (junction 80294)
            (junction 80295) -> (junction 80296) [order 1] : [PUSHED]
            (junction 80296) -> (junction 80297) [order 1] : [not(BUT_TEMP==FLOOR) || not(MOTION==2)]
            (junction 80297) -> Emergency.Doors.Closing3.Button_detection.Max_Min_assignment.MAX [order 1] : [MAX_BUT<BUT_TEMP && not(UPDATE)]
            (junction 80294) -> (junction 80299)
            (junction 80295) -> (junction 80309) [order 2]
            (junction 80296) -> (junction 80302) [order 2]
            (junction 80297) -> (junction 80298) [order 2]
            (junction 80299) -> (junction 80298)
            (junction 80298) -> (junction 80300)
            (junction 80300) -> Emergency.Doors.Closing3.Button_detection.Max_Min_assignment.MIN [order 1] : [MIN_BUT>BUT_TEMP && not(UPDATE)]
            Emergency.Doors.Closing3.Button_detection.Max_Min_assignment.MIN -> (junction 80301)
            (junction 80300) -> (junction 80303) [order 2]
            (junction 80301) -> (junction 80304)
            (junction 80303) -> (junction 80302)
            (junction 80304) -> (junction 80303)
            (junction 80302) -> (junction 80305)
            (junction 80305) -> Emergency.Doors.Closing3.Button_detection.Max_Min_assignment.Updating_button_0 [order 1] : [MOTION==0]
            Emergency.Doors.Closing3.Button_detection.Max_Min_assignment.Updating_button_0 -> (junction 80306)
            (junction 80305) -> (junction 80307) [order 2]
            (junction 80306) -> (junction 80308)
            (junction 80307) -> Emergency.Doors.Closing3.Button_detection.Max_Min_assignment.Updating_button_1 [order 1] : [MOTION==1]
            Emergency.Doors.Closing3.Button_detection.Max_Min_assignment.Updating_button_1 -> (junction 80308)
            (junction 80307) -> (junction 80310) [order 2]
            (junction 80308) -> (junction 80311)
            (junction 80310) -> (junction 80309)
            (junction 80311) -> (junction 80310)
          state GoTo_PositionControl
            en:
            BUTTON=BUT_TEMP;
            FLAG=2;
          state Emergency
            en:
            FLAG_EMG=true;
            FLAG=4;
          state Timer_EME
            state Set_tmr
              en:
              Q_EME=true;
            state Counting
              en:
              ET_EME= ET_EME + 1;
              Q_EME=false;
            state Set
              en:
              IN_EME=true;
              PT_EME=3;
            (junction 80401) -> Emergency.Doors.Closing3.Button_detection.Timer_EME.Set_tmr [order 1] : [ET_EME==PT_EME]
            Emergency.Doors.Closing3.Button_detection.Timer_EME.Set_tmr -> (junction 80402)
            Emergency.Doors.Closing3.Button_detection.Timer_EME.Counting -> (junction 80401)
            (junction 80401) -> (junction 80402) [order 2]
            (default) -> Emergency.Doors.Closing3.Button_detection.Timer_EME.Set
            Emergency.Doors.Closing3.Button_detection.Timer_EME.Set -> (junction 80403)
            (junction 80403) -> Emergency.Doors.Closing3.Button_detection.Timer_EME.Counting [order 1] : [ET_EME<PT_EME]
            (junction 80403) -> (junction 80402) [order 2]
          state Not_Emergency
            en:
            IN_EME=false;
            ET_EME=0;
          state SwitchingOFF_LEDs
            en:
            LPD3=false;
            LPD2=false;
            LPS2=false;
            LPD1=false;
            LPS1=false;
            LPS0=false;
          (default) -> (junction 80002)
          (junction 80002) -> (junction 80003) [order 1] : [FLAG==1 && not(PUSHED)]
              | {BUTTON=FLOOR;
              | BUT_TEMP=BUTTON;
              | BUT_1=FLOOR;}
          (junction 80003) -> Emergency.Doors.Closing3.Button_detection.Timer_LL [order 1] : [not(FLAG_STOP)]
          Emergency.Doors.Closing3.Button_detection.Save_energy -> (junction 80004)
          Emergency.Doors.Closing3.Button_detection.Timer_LL -> Emergency.Doors.Closing3.Button_detection.Save_energy
          (junction 80003) -> (junction 80006) [order 2]
          (junction 80002) -> (junction 80005) [order 2]
          (junction 80004) -> (junction 80007)
          (junction 80006) -> (junction 80005)
          (junction 80007) -> (junction 80006)
          (junction 80005) -> Emergency.Doors.Closing3.Button_detection.BUTTON_CAR
          Emergency.Doors.Closing3.Button_detection.BUTTON_UP -> Emergency.Doors.Closing3.Button_detection.BUTTON_DOWN
          Emergency.Doors.Closing3.Button_detection.BUTTON_DOWN -> Emergency.Doors.Closing3.Button_detection.Max_Min_assignment
          Emergency.Doors.Closing3.Button_detection.Max_Min_assignment -> (junction 80008)
          Emergency.Doors.Closing3.Button_detection.BUTTON_CAR -> Emergency.Doors.Closing3.Button_detection.BUTTON_UP
          (junction 80008) -> (junction 80010)
          (junction 80010) -> (junction 80009)
          (junction 80009) -> (junction 80012)
          Emergency.Doors.Closing3.Button_detection.GoTo_PositionControl -> (junction 80011)
          (junction 80012) -> (junction 80013) [order 1] : [FLAG==1]
          (junction 80013) -> Emergency.Doors.Closing3.Button_detection.GoTo_PositionControl [order 1] : [PUSHED]
          (junction 80011) -> (junction 80015)
          (junction 80012) -> (junction 80023) [order 2]
          (junction 80013) -> (junction 80014) [order 2]
          (junction 80015) -> (junction 80014)
          (junction 80014) -> (junction 80017)
          Emergency.Doors.Closing3.Button_detection.Emergency -> (junction 80016)
          (junction 80017) -> Emergency.Doors.Closing3.Button_detection.Timer_EME [order 1] : [STOP]
              | {IN_LL=false; ET_LL=0;FLAG=1;}
          Emergency.Doors.Closing3.Button_detection.Timer_EME -> (junction 80018)
          (junction 80018) -> Emergency.Doors.Closing3.Button_detection.Emergency [order 1] : [Q_EME]
          (junction 80016) -> (junction 80020)
          (junction 80017) -> Emergency.Doors.Closing3.Button_detection.Not_Emergency [order 2]
          (junction 80018) -> (junction 80019) [order 2]
          (junction 80020) -> (junction 80019)
          (junction 80019) -> (junction 80022)
          Emergency.Doors.Closing3.Button_detection.Not_Emergency -> (junction 80022)
          Emergency.Doors.Closing3.Button_detection.SwitchingOFF_LEDs -> (junction 80021)
          (junction 80022) -> Emergency.Doors.Closing3.Button_detection.SwitchingOFF_LEDs [order 1] : [FLAG_STOP && FLAG==2]
          (junction 80021) -> (junction 80025)
          (junction 80022) -> (junction 80024) [order 2]
          (junction 80024) -> (junction 80023)
          (junction 80025) -> (junction 80024)
        state Extending
          en:
          EXTEND=true;
        state Stop_Closing
          en:
          CP2=false;
          FLAG_OD=false;
          OBS=false;
          ET_cl=0;
          IN_cl=false;
        state GoTo_PositionControl
          en: FLAG=2;
        state GoTo_BUttonDetection
          en:
          MOTION=2;
          MAX_BUT=0;
          MIN_BUT=3;
          PUSHED=false;
          FIRST_BUT=true;
          FLAG=1;
          UPDATE=false;
        state Closing1
          en:CP2=true;
        state Stop_Closing1
          en:CP2=false;
        Emergency.Doors.Closing3.Reset -> Emergency.Doors.Closing3.Timer_close
        (default) -> (junction 79913)
        (junction 79913) -> Emergency.Doors.Closing3.Reset [order 1] : [not(FLAG==0) && not(FLAG==4)]
        Emergency.Doors.Closing3.Timer_close -> (junction 79914)
        (junction 79914) -> Emergency.Doors.Closing3.Closing [order 1] : [not(PC2)]
        Emergency.Doors.Closing3.Button_detection -> (junction 79915)
        Emergency.Doors.Closing3.Closing -> Emergency.Doors.Closing3.Button_detection
        (junction 79913) -> (junction 79923) [order 2]
        (junction 79914) -> (junction 79916) [order 2]
        (junction 79915) -> (junction 79921)
        (junction 79916) -> Emergency.Doors.Closing3.Extending [order 1] : [BUTTON==FLOOR]
        (junction 79916) -> (junction 79918) [order 2]
        Emergency.Doors.Closing3.Extending -> (junction 79917)
        (junction 79917) -> (junction 79918)
        (junction 79918) -> Emergency.Doors.Closing3.Stop_Closing
        Emergency.Doors.Closing3.Stop_Closing -> (junction 79919)
        (junction 79919) -> Emergency.Doors.Closing3.GoTo_PositionControl [order 2]
        (junction 79919) -> Emergency.Doors.Closing3.GoTo_BUttonDetection [order 1] : [not(BUTTON_CAR(1) || BUTTON_CAR(2) || BUTTON_CAR(3) || BUTTON_CAR(4) || BUTTON_UP(1) || BUTTON_UP(2) || BUTTON_UP(3) || BUTTON_DOWN(2) || BUTTON_DOWN(3) || BUTTON_DOWN(4))]
        Emergency.Doors.Closing3.GoTo_PositionControl -> (junction 79920)
        Emergency.Doors.Closing3.GoTo_BUttonDetection -> (junction 79920)
        (junction 79920) -> (junction 79921)
        (junction 79921) -> (junction 79922)
        (junction 79922) -> (junction 79924)
        (junction 79923) -> Emergency.Doors.Closing3.Closing1 [order 1] : [not(PC2)]
        Emergency.Doors.Closing3.Closing1 -> (junction 79924)
        (junction 79923) -> Emergency.Doors.Closing3.Stop_Closing1 [order 2]
        Emergency.Doors.Closing3.Stop_Closing1 -> (junction 79924)
      FLOOR_0 -> Emergency.Doors.Opening0
      (junction 15604) -> (junction 15603) [order 1] : [(SWITCH || FLAG_EMG || FLAG_BO) && (RPC0 || RPC1 || RPC2 || RPC3)]
      (junction 15603) -> FLOOR_0 [order 1] : [FLOOR==0]
      Emergency.Doors.Opening0 -> (junction 36735)
      (default) -> (junction 15604)
      (junction 15604) -> (junction 36752) [order 2]
      (junction 15603) -> (junction 36727) [order 2]
      (junction 36735) -> (junction 36737)
      FLOOR_1 -> Emergency.Doors.Opening1
      (junction 36727) -> FLOOR_1 [order 1] : [FLOOR==1]
      Emergency.Doors.Opening1 -> (junction 36737)
      (junction 36727) -> (junction 36730) [order 2]
      (junction 36737) -> (junction 36741)
      FLOOR_2 -> Emergency.Doors.Opening2
      (junction 36730) -> FLOOR_2 [order 1] : [FLOOR==2]
      Emergency.Doors.Opening2 -> (junction 36741)
      (junction 36730) -> (junction 36732) [order 2]
      (junction 36741) -> (junction 36744)
      FLOOR_3 -> Emergency.Doors.Opening3
      Emergency.Doors.Opening3 -> (junction 36744)
      (junction 36732) -> FLOOR_3 [order 1] : [FLOOR==3]
      (junction 36744) -> (junction 36749)
      (junction 36732) -> (junction 36747) [order 2]
      (junction 36747) -> (junction 36752)
      (junction 36749) -> (junction 36747)
      (junction 36752) -> (junction 36755)
      (junction 36755) -> (junction 15605) [order 1] : [not(BO) && FLAG_OD && not(FLAG_EMG)]
      (junction 15605) -> Emergency.Doors.Closing0 [order 1] : [FLOOR==0]
      Emergency.Doors.Closing0 -> (junction 36764)
      (junction 36755) -> (junction 36780) [order 2]
      (junction 15605) -> (junction 36757) [order 2]
      (junction 36764) -> (junction 36766)
      (junction 36757) -> Emergency.Doors.Closing1 [order 1] : [FLOOR==1]
      Emergency.Doors.Closing1 -> (junction 36766)
      (junction 36757) -> (junction 36759) [order 2]
      (junction 36766) -> (junction 36767)
      Emergency.Doors.Closing2 -> (junction 36767)
      (junction 36759) -> Emergency.Doors.Closing2 [order 1] : [FLOOR==2]
      (junction 36767) -> (junction 36768)
      (junction 36759) -> (junction 36761) [order 2]
      (junction 36761) -> Emergency.Doors.Closing3 [order 1] : [FLOOR==3]
      Emergency.Doors.Closing3 -> (junction 36768)
      (junction 36761) -> (junction 36763) [order 2]
      (junction 36768) -> (junction 36769)
      (junction 36763) -> (junction 36780)
      (junction 36769) -> (junction 36763)
    state Timer_EME_OFF
      state Set_tmr
        en: Q_EME_OFF=true;
      state Counting
        en:ET_EME_OFF = ET_EME_OFF + 1;
        Q_EME_OFF=false;
      state Set
        en:PT_EME_OFF=3;
        IN_EME_OFF=true;
      (junction 16326) -> Emergency.Timer_EME_OFF.Set_tmr [order 1] : [ET_EME_OFF==PT_EME_OFF]
      Emergency.Timer_EME_OFF.Set_tmr -> (junction 16327)
      Emergency.Timer_EME_OFF.Counting -> (junction 16326)
      (junction 16326) -> (junction 16327) [order 2]
      (default) -> Emergency.Timer_EME_OFF.Set
      Emergency.Timer_EME_OFF.Set -> (junction 16328)
      (junction 16328) -> Emergency.Timer_EME_OFF.Counting [order 1] : [ET_EME_OFF<PT_EME_OFF]
      (junction 16328) -> (junction 16327) [order 2]
    state NOT_EME
      en:
      FLAG_EMG=false;
    state KEEP_EME
      en:
      IN_EME_OFF=false;
      ET_EME_OFF=0;
    state NOT_BO
      en:
      FLAG_BO=false;
    state EME_FINISH
      en:
      FLAG=1;
      LPS0=false; LPS1=false;
      LPD1=false; LPS2=false;
      LPD2=false; LPD3=false;
      OBS=false; FLAG_OD=false;
      IN_cl=false; ET_cl=0;
      IN_EME=false; ET_EME=0;
      IN_EME_OFF=false; ET_EME_OFF=0;
      FIRST=true; FLAG_REC=false;
      PUSHED=false;
      MAX_BUT=0; MIN_BUT=3;
    (junction 36672) -> BLK_Eme [order 1] : [FLAG_EMG]
    (default) -> (junction 36672)
    (junction 36672) -> (junction 36674) [order 2]
    BLK_Eme -> (junction 36675)
    (junction 36674) -> (junction 36675)
    (junction 36675) -> REC [order 1] : [FLAG_REC && BO]
    (junction 36675) -> (junction 36682) [order 2]
    REC -> (junction 36681)
    (junction 36682) -> (junction 36681)
    (junction 36681) -> FIRST [order 1] : [FIRST]
    (junction 36681) -> (junction 36687) [order 2]
    FIRST -> (junction 36686)
    (junction 36687) -> (junction 36686)
    (junction 36686) -> Emergency.Replacing [order 1] : [not(RPC0) && not(RPC1) && not(RPC2) && not(RPC3)]
    (junction 36686) -> Emergency.Replaced [order 2]
    Emergency.Replacing -> (junction 36692)
    Emergency.Replaced -> (junction 36691)
    Doors -> (junction 36697)
    (junction 36691) -> Doors
    (junction 36692) -> (junction 36691)
    (junction 36697) -> (junction 36699)
    (junction 36699) -> (junction 15583) [order 1] : [((not(BO) && not(FLAG_REC)) || FLAG_EMG) && not(FIRE)]
    (junction 15583) -> Timer_EME_OFF [order 1] : [STOP && (PA0 || PA1|| PA2 || PA3)]
    Timer_EME_OFF -> (junction 36701)
    (junction 36701) -> NOT_EME [order 1] : [Q_EME_OFF]
    (junction 36699) -> (junction 36711) [order 2]
    (junction 15583) -> KEEP_EME [order 2]
    (junction 36701) -> (junction 36703) [order 2]
    NOT_EME -> (junction 36705)
    KEEP_EME -> (junction 36708)
    (junction 36708) -> (junction 36711)
    (junction 36703) -> (junction 36708)
    (junction 36705) -> (junction 36703)
    (junction 36711) -> (junction 36714)
    (junction 36714) -> NOT_BO [order 1] : [(PA0 || PA1 || PA2 || PA3) && not(BO)]
    (junction 36714) -> (junction 36719) [order 2]
    NOT_BO -> (junction 36716)
    (junction 36719) -> (junction 36716)
    (junction 36716) -> EME_FINISH [order 1] : [(RPC0 || RPC1 || RPC2 || RPC3) && (PC0 && PC1 && PC2 && PC3) && not(FLAG_EMG) && not (BO)]
    (junction 36716) -> (junction 36722) [order 2]
    EME_FINISH -> (junction 36723)
    (junction 36723) -> (junction 36722)
  Init_procedure -> (junction 26970)
  (default) -> Blackout
  Blackout -> Fire_detection
  Fire_detection -> Floor_detection
  Floor_detection -> (junction 4471)
  (junction 4471) -> Init_procedure [order 1] : [FLAG==0]
  (junction 26970) -> (junction 26972)
  (junction 4471) -> (junction 26959) [order 2]
  (junction 26984) -> Blackout
  (junction 26959) -> Button_detection [order 1] : [FLAG==1]
  Button_detection -> (junction 26972)
  (junction 26959) -> (junction 26961) [order 2]
  (junction 26972) -> (junction 26975)
  (junction 26961) -> Position_control [order 1] : [FLAG==2]
  Position_control -> (junction 26975)
  (junction 26961) -> (junction 26963) [order 2]
  (junction 26975) -> (junction 26978)
  OpCl_doors -> (junction 26978)
  (junction 26963) -> OpCl_doors [order 1] : [FLAG==3]
  (junction 26978) -> (junction 26981)
  (junction 26963) -> (junction 26965) [order 2]
  (junction 26965) -> Emergency [order 1] : [FLAG==4]
  Emergency -> (junction 26981)
  (junction 26965) -> (junction 26984) [order 2]
  (junction 26981) -> (junction 27112)
  (junction 27112) -> (junction 26984)
  data: FLAG local =0; STOP input boolean =false; BUTTON local =0; FLOOR local =0; SALI output =false; SCENDI output =false; PS1 input; PD1 input; P1 input; PD2 input; PS2 input; P2 input; PD3 input; P3 input; PS0 input; SWITCH input; P0 input; LPC3 output =false; LPC1 output =false; LPC0 output =false; LPC2 output =false; RPC2 input; RPC1 input; RPC3 input; RPC0 input; AP1 output =false; LPS0 output =false; LPS1 output =false; LPS2 output =false; CP3 output =false; LPD2 output =false; LPD1 output =false; LPD3 output =false; CP1 output =false; AP0 output =false; CP0 output =false; AP2 output =false; CP2 output =false; AP3 output =false; OBS local =false; FLAG_OD local =false; PC3 input; PC2 input; PC0 input; PC1 input; PA3 input; PA1 input; PA2 input; PA0 input; IN_LL local =false; IN_EME local =false; IN_op local =false; IN_EME_OFF local =false; IN_cl local =false; FIRST local =false; FLAG_BO local =false; BUT_TEMP local =0; Q_op local =false; PT_cl local; LL output =false; Q_LL local =false; ET_LL local =0; PT_LL local =0; Q_EME local =false; ET_EME local =0; PT_EME local =0; MOTION local =0; PT_op local =0; ET_EME_OFF local =0; FLAG_STOP local =false; Q_EME_OFF local =false; PT_EME_OFF local =0; ET_op local =0; WOMEN local =0; WEIGHT local =0; ET_cl local =0; FATGUYS local =0; Q_cl local =false; MEN local =0; KIDS local =0; COUNTER_IN local =false; COUNTER_OUT local =false; FLAG_REC local =false; FLAG_EMG local =false; RECOVERY local =false; BO local =false; FIRE local =false; MAN_OUT local =false; WOMAN_IN local =false; MAN_IN local =false; KID_IN local =false; KID_OUT local =false; WOMAN_OUT local =false; FATGUY_OUT local =false; FATGUY_IN local =false; BUTTON_CAR local boolean size=[1,4] =[false false false false]; BUTTON_UP local boolean size=[1,4] =[false false false false]; FIRST_BUT local =false; BUTTON_DOWN local boolean size=[1,4] =[false false false false]; MOTION_TEMP local =0; BUT_1 local =0; MIN_BUT local =0; UPDATE local =false; PUSHED local =false; MAX_BUT local =0; EXTEND local =false
